simulink model "empty"  (Simulink 7.9)
settings: Solver=ode15s  StartTime=0.0  StopTime=10*24*3600  RelTol=1e-3
undefined symbols (not defined in the file): B, U, x0
settings Model: Creator=M.Sparnaaij  LastModifiedBy=M.Sparnaaij  ExtModeTrigMode=oneshot  ExtModeArmWhenConnect=off
settings DataIOCC: LimitDataPoints=off  SignalLoggingName=sigsOut
settings OptimizationCC: BooleanDataType=off
settings DebuggingCC: SaveWithParameterizedLinksMsg=none  SignalResolutionControl=TryResolveAllWithWarning  SolverPrmCheckMsg=none  MultiTaskDSMMsg=warning  MultiTaskCondExecSysMsg=none  StrictBusMsg=None
settings HardwareCC: TargetUnknown=on
settings RTWCC: IncludeERTFirstTime=on
settings GRTTargetCC: CombineOutputUpdateFcns=off  GRTInterface=on

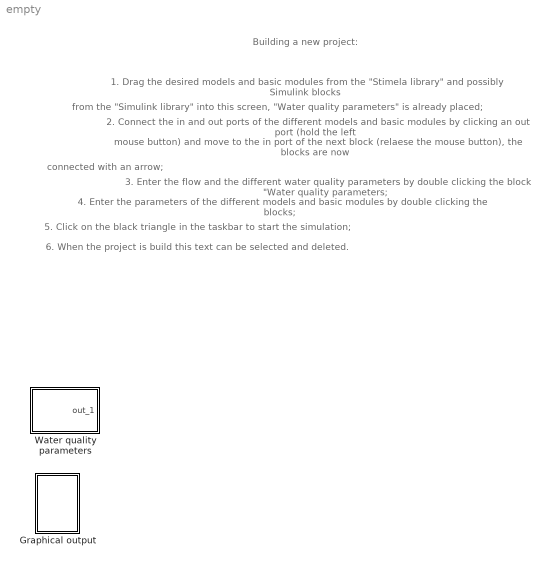
== system empty ==
  note: 1. Drag the desired models and basic modules from the "Stimela library" and possibly Simulink blocks
  note: 2. Connect the in and out ports of the different models and basic modules by clicking an out port (hold the left
  note: mouse button) and move to the in port of the next block (relaese the mouse button), the blocks are now
  note: connected with an arrow;
  note: from the "Simulink library" into this screen, "Water quality parameters" is already placed;
  note: 3. Enter the flow and the different water quality parameters by double clicking the block "Water quality parameters;
  note: 4. Enter the parameters of the different models and basic modules by double clicking the blocks;
  note: Building a new project:
  note: 6. When the project is build this text can be selected and deleted.
  note: 5. Click on the black triangle in the taskbar to start the simulation;
  Graphical output : Subsystem
      settings: OpenFcn=plotStimela2
      mask Display:
      | plot(0,0,100,100,[80,20,20],[20,20,80],[80,69,60,52,45,39,33,28,24,20],[65,65,64,61,57,52,45,37,30,20])
      | disp('');
      | text(100,100,'Stimela', 'horizontalAlignment', 'right', 'verticalAlignment', 'top');
  Water quality parameters : Subsystem  Description=The water flow and the water quality data must be filled out in the 'Water quality parameters' block. Each project must start with a 'Water quality parameters' block.
      mask init:
      | filenaam='./StimelaData/rawwater.mat';
      | 
      | [Pn,Fn,Fext]=Fileprop(filenaam);
      | 
      | errstr = st_UniqName(filenaam,'filenaam=''','SubSystem','OpenFcn');
      | if errstr, error([errstr 'The filename "' filenaam '" is already in use. Choose a different filename.']), end
      | 
      | P = invruw_p(filenaam);
      | [B,x0,U]=invruw_i(filenaam);
      settings: OpenFcn=|
      | filenaam='./StimelaData/rawwater.mat';
      | st_ParameterInput('init',gcb,filenaam,'invruw');
      mask Display:
      | plot(0,0,100,100,[80 100],[ 50 50],[80 100],[ 55 55],[20 80 80 20 20],[10 10 90  90 10]);
      | disp('')
      | text(50,50,'invruw', 'horizontalAlignment', 'center', 'verticalAlignment', 'middle');
      | text(50,0,Fn, 'horizontalAlignment', 'center', 'verticalAlignment', 'base');

== system empty/Graphical output ==
  note: plotten

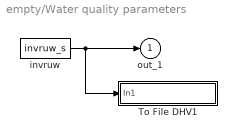
== system empty/Water quality parameters ==
  To File DHV1 : Subsystem  mask(To File DHV){naam=[filenaam(1:length(filenaam)-4) '_out.sti']}
      mask prompts: naam "Naam van bestand"
      mask init:
      | set_param([gcb '/To File'],'Filename',naam);
      mask Display: disp(naam)
  invruw : S-Function  FunctionName=invruw_s  Parameters=B,x0,U,P  EnableBusSupport=off
  out_1 : Outport  InitialOutput=0
  wires:
  invruw/1 -> out_1/1, To File DHV1/1(In1)

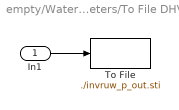
== system empty/Water quality parameters/To File DHV1 ==
  In1 : Inport
  To File : ToFile  Filename=./invruw_p_out.sti  MatrixName=invruwout
  wires:
  In1/1 -> To File/1
